simulink model "fi_2_worksp"  (Simulink 7.8)
settings: Solver=FixedStepDiscrete  StartTime=0.0  StopTime=100  RelTol=1e-3
values from neighbouring files (symbols this model uses):
  Ts = 1/fs    (= 6.25e-05)    [G722_1.m]    (also in adaptiv_2.m = 0.001; adaptiv_3.m = 0.001; adaptiv_4.m = 0.001; adaptiv_5.m = 0.001)
undefined symbols (not defined in the file or in its folder): dfilt
libraries: dspsigops x1, dsparch4 x1
settings Model: MinMaxOverflowLogging=MinMaxAndOverflow  Creator=svenhoffmann  LastModifiedBy=josef  ExtModeAutoUpdateStatusClock=off
settings OptimizationCC: InitFltsAndDblsToZero=on
settings DebuggingCC: SaveWithParameterizedLinksMsg=none  SignalResolutionControl=TryResolveAllWithWarning  MultiTaskDSMMsg=warning  MultiTaskCondExecSysMsg=none  FcnCallInpInsideContextMsg=Use local settings  StrictBusMsg=Warning
settings RTWCC: IncludeERTFirstTime=on
settings GRTTargetCC: TargetFcnLib=ansi_tfl_tmw.mat

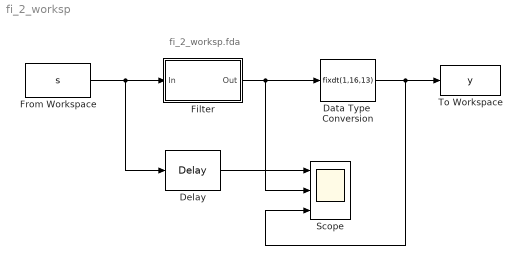
== system fi_2_worksp ==
  note: fi_2_worksp.fda
  Data Type  Conversion : DataTypeConversion  OutDataTypeStr=fixdt(1,16,13)  SaturateOnIntegerOverflow=on  RndMeth=Zero
  Delay : dspsigops/Delay  InputProcessing=Inherited (this choice will be removed - see release notes)  dly_unit=Samples  delay=50  ic_detail=off  dif_ic_for_ch=off  dif_ic_for_dly=off  ic=0  reset_popup=None
  Filter : Subsystem  Tag=BlockMethodSubSystem
  From Workspace : FromWorkspace  VariableName=s  SampleTime=Ts  Interpolate=off  OutputAfterFinalValue=Holding final value
  Scope : Scope  NumInputPorts=3
      settings: YMin=-5~-5~-5  YMax=5~5~5
  To Workspace : ToWorkspace  VariableName=y  SampleTime=-1  SaveFormat=Structure
  wires:
  From Workspace/1 -> Filter/1(In), Delay/1
  Filter/1(Out) -> Data Type  Conversion/1, Scope/2
  Delay/1 -> Scope/1
  Data Type  Conversion/1 -> To Workspace/1, Scope/3

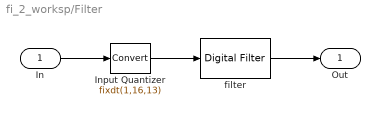
== system fi_2_worksp/Filter ==
  In : Inport
  Input Quantizer : DataTypeConversion  OutDataTypeStr=fixdt(1,16,13)  RndMeth=Round  SaturateOnIntegerOverflow=on
  filter : dsparch4/Digital Filter  TypePopup=FIR (all zeros)  IIRFiltStruct=Direct form II transposed  AllPoleFiltStruct=Direct form  FIRFiltStruct=Direct form  CoeffSource=Specify via dialog  NumCoeffs=[-0.000219289468611461 -0.00049003386170769 -0.000824439948465002 -0.00102637985561707 -0.000834895235538483 6.09651389453232e-06 0.00161877298313516 0.00386715020949695 0.00630295230152784 0.00823418387240124 0.00892822924454265 0.00789649310235671 0.00515640806304935 0.00134413745500198 -0.00240856686292956 -0.00483425577988972 -0.00501850890997209 -0.00282654976130475 0.000931215853242073 0.00471503472683744 0.00682139629282983 0.00610247136510244 0.00254151024032591 -0.00259567297125691 -0.00716457438605087 -0.00899868002063117 -0.00689426755474144 -0.00129353098886089 0.0056892232886382 0.0110036876529725 0.0119337967496587 0.00739781225648747 -0.00131118902056871 -0.0107631601224708 -0.0166420438801746 -0.015592101326238 -0.00691533930765561 0.00666354579504925 0.0196470140271202 0.0257608721832168 0.0206362962732825 0.00413515769041731 -0.0187095652623527 -0.0387220727436496 -0.0454316254847004 -0.0308452257626461 0.00720472870007785 0.0634465099028758 0.126042315140226 0.17982017744595 0.210855562552222 0.210855562552222 0.17982017744595 0.126042315140226 0.0634465099028758 0.00720472870007785 -0.0308452257626461 -0.0454316254847004 -0.0387220727436496 -0.0187095652623527 0.00413515769041731 0.0206362962732825 0.0257608721832168 0.0196470140271202 0.00666354579504925 -0.00691533930765561 -0.015592101326238 -0.0166420438801746 -0.0107631601224708 -0.00131118902056871 0.00739781225648747 0.0119337967496587 0.0110036876529725 0.0056892232886382 -0.00129353098886089 -0.00689426755474144 -0.00899868002063117 -0.00716457438605087 -0.00259567297125691 0.00254151024032591 0.00610247136510244 0.00682139629282983 0.00471503472683744 0.000931215853242073 -0.00282654976130475 -0.00501850890997209 -0.00483425577988972 -0.00240856686292956 0.00134413745500198 0.00515640806304935 0.00789649310235671 0.00892822924454265 0.00823418387240124 0.00630295230152784 0.00386715020949695 0.00161877298313516 6.09651389453232e-06 -0.000834895235538483 -0.00102637985561707 -0.000824439948465002 -0.00049003386170769 -0.000219289468611461]  DenCoeffs=[1 0.1]  BiQuadCoeffs=[1 0.3 0.4 1 0.1 0.2]  LatticeCoeffs=[0.2 0.4]  denIgnore=on  FiltPerSampPopup=One filter per frame  IC=0  ICnum=0  ICden=0  firstCoeffMode=Binary point scaling  firstCoeffWordLength=16  firstCoeffFracLength=17  outputMode=Binary point scaling  outputWordLength=34  outputFracLength=30  accumMode=Binary point scaling  accumWordLength=34  accumFracLength=30  prodOutputMode=Binary point scaling  prodOutputWordLength=31  prodOutputFracLength=30  roundingMode=Convergent  overflowMode=off  ScaleValues=1  scaleValueFracLength=14  stageInFracLength=15  stageOutFracLength=15  FilterSource=Specify via dialog  dfiltObjectName=dfilt.dffir([1 2 1])  InputProcessing=Columns as channels (frame based)
  Out : Outport
  wires:
  In/1 -> Input Quantizer/1
  Input Quantizer/1 -> filter/1
  filter/1 -> Out/1
